simulink model "MOCS_AS_Gen"  (R2022b)
settings: Solver=FixedStepDiscrete  StartTime=0.0  StopTime=inf  FixedStep=0.1  RelTol=1e-3
undefined symbols (not defined in the file): CommonReservedCat2_typ, FODS_typ, FODSFeedback_typ, FODSFeedforward_typ, IF_PARA_CFlag, IF_PARA_CFODS, IF_PARA_CMain, IF_PARA_CReserved, IF_PARA_CSys, IF_PARA_No1FB, IF_PARA_No1FF, IF_PARA_No1Reserved, IF_PARA_No2FB, IF_PARA_No2FF, IF_PARA_No2Reserved, IF_PARA_No3FB, IF_PARA_No3FF, IF_PARA_No3Reserved, IF_PARA_No4FB, IF_PARA_No4FF, IF_PARA_No4Reserved, IF_PARA_No5FB, IF_PARA_No5FF, IF_PARA_No5Reserved, IF_PARA_No6FB, IF_PARA_No6FF, IF_PARA_No6Reserved, IF_PARA_No7FB, IF_PARA_No7FF, IF_PARA_No7Reserved, IF_PARA_No8FB, IF_PARA_No8FF, IF_PARA_No8Reserved, IndivReservedCat2_typ, Main_typ, StateFlag_typ, System_typ
libraries: bur_blks x39
settings Model: Creator=HHI  LastModifiedBy=HHI
settings DataIOCC: SaveFormat=Array  SaveOutput=off  SignalLogging=off  DSMLogging=off  SaveTime=off  ReturnWorkspaceOutputs=off
settings OptimizationCC: EnableMemcpy=off  ZeroExternalMemoryAtStartup=off  ZeroInternalMemoryAtStartup=off  InitFltsAndDblsToZero=on  LifeSpan=inf  OptimizeBlockOrder=speed  DifferentSizesBufferReuse=on  EfficientTunableParamExpr=on
settings DebuggingCC: UnderspecifiedInitializationDetection=Classic  MergeDetectMultiDrivingBlocksExec=none  SolverPrmCheckMsg=warning  InheritedTsInSrcMsg=none  FcnCallInpInsideContextMsg=warning  UnconnectedInputMsg=warning  UnconnectedOutputMsg=warning  UnconnectedLineMsg=warning  FrameProcessingCompatibilityMsg=none  ModelReferenceSymbolNameMessage=none  StateNameClashWarn=warning  SFUnexpectedBacktrackingDiag=warning  SFNoUnconditionalDefaultTransitionDiag=warning
settings HardwareCC: ProdBitPerPointer=32  ProdBitPerSizeT=32  ProdBitPerPtrDiffT=32  ProdLargestAtomicFloat=None  ProdWordSize=32  ProdHWDeviceType=Intel->x86/Pentium
settings ModelReferenceCC: UpdateModelReferenceTargets=IfOutOfDate  ModelReferencePassRootInputsByReference=off  PropagateSignalLabelsOutOfModel=off
settings SFSimCC: MATLABDynamicMemAlloc=off
settings RTWCC: Description=B&R Automation Studio Target (ERT based)  SystemTargetFile=bur_ert.tlc  GenCodeOnly=on  GenerateMakefile=off  TemplateMakefile=bur.tmf  RTWVerbose=off
settings CodeAppCC: IgnoreTestpoints=on  CustomSymbolStrType=$N$R$M  InternalIdentifier=Classic
settings STFCustomTargetCC: TargetLangStandard=C99 (ISO)  MultiwordLength=256  ParMdlRefBuildCompliant=on  ERTCustomFileBanners=on  SupportNonFinite=off  SupportNonInlinedSFcns=off  RemoveResetFunc=on  MATLABClassNameForMDSCustomization=Simulink.SoftwareTarget.ERTCustomization  SystemTargetFile=bur_ert.tlc
settings ERTTargetCC: TargetLangStandard=C99 (ISO)  CompOptLevelCompliant=off  ConcurrentExecutionCompliant=off  CombineOutputUpdateFcns=off  SupportNonFinite=off  SupportContinuousTime=on  ModelStepFunctionPrototypeControlCompliant=off  CPPClassGenCompliant=off  UseToolchainInfoCompliant=off  ExtModeMexArgs='127.0.0.1'  MultiInstanceErrorCode=Warning  RootIOFormat=Structure reference  ERTSrcFileBannerTemplate=bur_code_c_template.cgt  ERTHdrFileBannerTemplate=bur_code_h_template.cgt  ERTDataSrcFileTemplate=bur_data_c_template.cgt  ERTDataHdrFileTemplate=bur_data_h_template.cgt  ERTCustomFileTemplate=bur_file_process.tlc  ConvertIfToSwitch=off  SuppressUnreachableDefaultCases=off

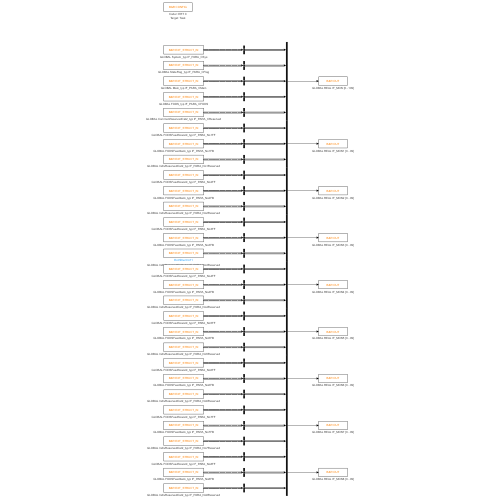
[thumbnail: Simulink's stored preview of the top-level diagram]
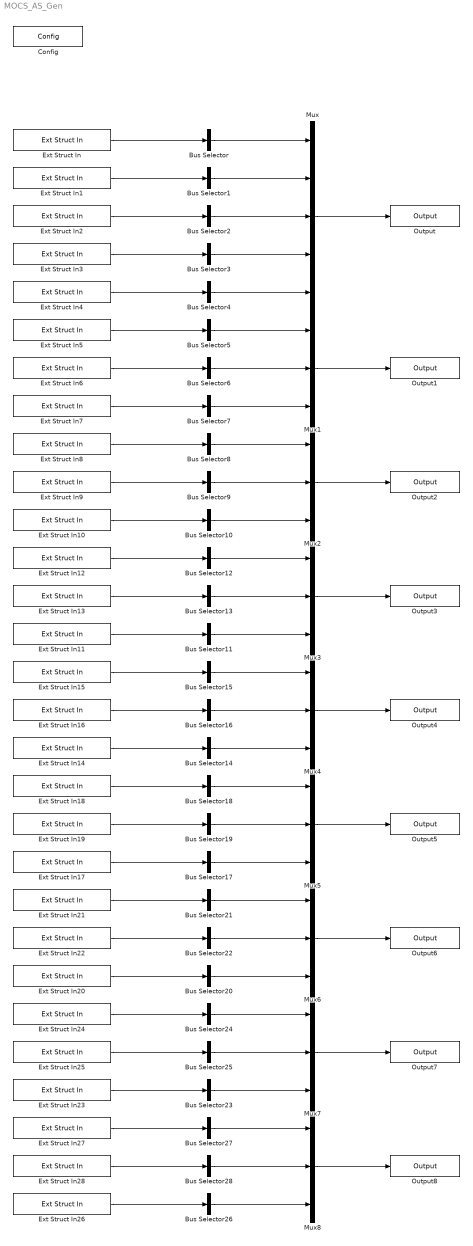
== system MOCS_AS_Gen ==
  Bus Selector : BusSelector  OutputSignals=SystemType.MOCSType,SystemType.NumofGE,SystemType.HeatingSystem,SystemType.FOSuppUnit,SystemReserved.SystemReserved4,SystemReserved.SystemReserved5,SystemReserved.SystemReserved6,SystemReserved.SystemReserved7,SystemReserved.SystemReserved8,SystemReserved.SystemReserved9,SystemReserved.SystemReserved10,SystemReserved.SystemReserved11,SystemReserved.SystemReserved12,SystemReserved.SystemReserved13,SystemReserved.SystemReserved14,SystemReserved.SystemReserved15,SystemReserved.SystemReserved16,SystemReserved.SystemReserved17,SystemReserved.SystemReserved18,SystemReserved.SystemReserved19,SystemReserved.SystemReserved20,SystemReserved.SystemReserved21,SystemReserved.SystemReserved22,SystemReserved.SystemReserved23,SystemReserved.SystemReserved24,SystemReserved.SystemReserved25,SystemReserved.SystemReserved26,SystemReserved.SystemReserved27,SystemReserved.SystemReserved28,SystemReserved.SystemReserved29,SystemReserved.SystemReserved30,SystemReserved.SystemReserved31,SystemReserved.SystemReserved32,SystemReserved.SystemReserved33,SystemReserved.SystemReserved34,SystemReserved.SystemReserved35,SystemReserved.SystemReserved36,SystemReserved.SystemReserved37,SystemReserved.SystemReserved38,SystemReserved.SystemReserved39,SystemReserved.SystemReserved40,SystemReserved.SystemReserved41,SystemReserved.SystemReserved42,SystemReserved.SystemReserved43,SystemReserved.SystemReserved44,SystemReserved.SystemReserved45,SystemReserved.SystemReserved46,SystemReserved.SystemReserved47,SystemReserved.SystemReserved48,SystemReserved.SystemReserved49  OutputAsBus=on
  Bus Selector1 : BusSelector  OutputSignals=MSSNormalFlag.MOCSMinEngineLoad,MSSNormalFlag.MOCSReadyEngineLoad,MSSNormalFlag.MSSNormalFallingHysteresis,MSSNormalFlag.MSSNormalFallingDelay,MSSNormalFlag.MSSFlagReserved4,LoadChangeFlag.MovAvgPeriod,LoadChangeFlag.ComparePoint,LoadChangeFlag.LoadChangeThreshold,LoadChangeFlag.TMBFlagFallingDelay,LoadChangeFlag.TMBFlagReserved4,SystemWarmedUpFlag.WarmUpDTemp,SystemWarmedUpFlag.WarmUpITemp,SystemWarmedUpFlag.WarmUpChITemp,SystemWarmedUpFlag.WarmUpChMTemp,SystemWarmedUpFlag.WarmUpChOTemp,FlagReserved.FlagReserved15,FlagReserved.FlagReserved16,FlagReserved.FlagReserved17,FlagReserved.FlagReserved18,FlagReserved.FlagReserved19,FlagReserved.FlagReserved20,FlagReserved.FlagReserved21,FlagReserved.FlagReserved22,FlagReserved.FlagReserved23,FlagReserved.FlagReserved24,FlagReserved.FlagReserved25,FlagReserved.FlagReserved26,FlagReserved.FlagReserved27,FlagReserved.FlagReserved28,FlagReserved.FlagReserved29,FlagReserved.FlagReserved30,FlagReserved.FlagReserved31,FlagReserved.FlagReserved32,FlagReserved.FlagReserved33,FlagReserved.FlagReserved34,FlagReserved.FlagReserved35,FlagReserved.FlagReserved36,FlagReserved.FlagReserved37,FlagReserved.FlagReserved38,FlagReserved.FlagReserved39,FlagReserved.FlagReserved40,FlagReserved.FlagReserved41,FlagReserved.FlagReserved42,FlagReserved.FlagReserved43,FlagReserved.FlagReserved44,FlagReserved.FlagReserved45,FlagReserved.FlagReserved46,FlagReserved.FlagReserved47,FlagReserved.FlagReserved48,FlagReserved.FlagReserved49  OutputAsBus=on
  Bus Selector{7,10..11,14,17,20,23,26} (8 alike) : BusSelector  OutputSignals=IndivReservedCat3.IndivReserved75,IndivReservedCat3.IndivReserved76,IndivReservedCat3.IndivReserved77,IndivReservedCat3.IndivReserved78,IndivReservedCat3.IndivReserved79,IndivReservedCat3.IndivReserved80,IndivReservedCat3.IndivReserved81,IndivReservedCat3.IndivReserved82,IndivReservedCat3.IndivReserved83,IndivReservedCat3.IndivReserved84,IndivReservedCat3.IndivReserved85,IndivReservedCat3.IndivReserved86,IndivReservedCat3.IndivReserved87,IndivReservedCat3.IndivReserved88,IndivReservedCat3.IndivReserved89,IndivReservedCat3.IndivReserved90,IndivReservedCat3.IndivReserved91,IndivReservedCat3.IndivReserved92,IndivReservedCat3.IndivReserved93,IndivReservedCat3.IndivReserved94,IndivReservedCat3.IndivReserved95,IndivReservedCat3.IndivReserved96,IndivReservedCat3.IndivReserved97,IndivReservedCat3.IndivReserved98,IndivReservedCat3.IndivReserved99  OutputAsBus=on
  Bus Selector{5,8,12,15,18,21,24,27} (8 alike) : BusSelector  OutputSignals=FFpara.NumTableRow,FFpara.HeatLossTemp,EngineLoad.EngineLoad0,EngineLoad.EngineLoad1,EngineLoad.EngineLoad2,EngineLoad.EngineLoad3,EngineLoad.EngineLoad4,EngineLoad.EngineLoad5,EngineLoad.EngineLoad6,EngineLoad.EngineLoad7,EngineLoad.EngineLoad8,EngineLoad.EngineLoad9,EngineLoad.EngineLoad10,EngineLoad.EngineLoad11,ExhFlowrate.ExhFlowrate0,ExhFlowrate.ExhFlowrate1,ExhFlowrate.ExhFlowrate2,ExhFlowrate.ExhFlowrate3,ExhFlowrate.ExhFlowrate4,ExhFlowrate.ExhFlowrate5,ExhFlowrate.ExhFlowrate6,ExhFlowrate.ExhFlowrate7,ExhFlowrate.ExhFlowrate8,ExhFlowrate.ExhFlowrate9,ExhFlowrate.ExhFlowrate10,ExhFlowrate.ExhFlowrate11,HUInletRefTemp.HUInletRefTemp0,HUInletRefTemp.HUInletRefTemp1,HUInletRefTemp.HUInletRefTemp2,HUInletRefTemp.HUInletRefTemp3,HUInletRefTemp.HUInletRefTemp4,HUInletRefTemp.HUInletRefTemp5,HUInletRefTemp.HUInletRefTemp6,HUInletRefTemp.HUInletRefTemp7,HUInletRefTemp.HUInletRefTemp8,HUInletRefTemp.HUInletRefTemp9,HUInletRefTemp.HUInletRefTemp10,HUInletRefTemp.HUInletRefTemp11,CorrectionFactor.CorrectionFactor0,CorrectionFactor.CorrectionFactor1,CorrectionFactor.CorrectionFactor2,CorrectionFactor.CorrectionFactor3,CorrectionFactor.CorrectionFactor4,CorrectionFactor.CorrectionFactor5,CorrectionFactor.CorrectionFactor6,CorrectionFactor.CorrectionFactor7,CorrectionFactor.CorrectionFactor8,CorrectionFactor.CorrectionFactor9,CorrectionFactor.CorrectionFactor10,CorrectionFactor.CorrectionFactor11  OutputAsBus=on
  Bus Selector{6,9,13,16,19,22,25,28} (8 alike) : BusSelector  OutputSignals=MOCSTempPgain.MOCSTempPgain0,MOCSTempPgain.MOCSTempPgain1,MOCSTempPgain.MOCSTempPgain2,MOCSTempPgain.MOCSTempPgain3,MOCSTempPgain.MOCSTempPgain4,MOCSTempPgain.MOCSTempPgain5,MOCSTempPgain.MOCSTempPgain6,MOCSTempPgain.MOCSTempPgain7,MOCSTempPgain.MOCSTempPgain8,MOCSTempPgain.MOCSTempPgain9,MOCSTempPgain.MOCSTempPgain10,MOCSTempPgain.MOCSTempPgain11,APIDgain.MOCSTempIgain,APIDgain.MOCSTempDgain,APIDgain.MOCSTempNoiseSup,APIDgain.QFOPgain,APIDgain.QFOIgain,APIDgain.QFODgain,APIDgain.QFONoiseSup,APIDgain.FODSFeedbackReserved19,APIDgain.FODSFeedbackReserved20,APIDgain.FODSFeedbackReserved21,APIDgain.FODSFeedbackReserved22,APIDgain.FODSFeedbackReserved23,APIDgain.FODSFeedbackReserved24  OutputAsBus=on
  Bus Selector2 : BusSelector  OutputSignals=Init.InitReserved0,Init.InitReserved1,Init.InitReserved2,Init.InitReserved3,Init.InitReserved4,Sealing.VSSolValveOpenDP,Sealing.VSSolValveCloseDP,Sealing.RTVOpenDP,Sealing.RTVCloseDP,Sealing.SealRTVSetpoint,Sealing.VSSolValveOpenDuration,Sealing.VSSolValveCloseDuration,Sealing.SealingReserved7,Sealing.SealingReserved8,Sealing.SealingReserved9,Engage.EnRTVSlope,Engage.EngageReserved1,Engage.EngageReserved2,Engage.EngageReserved3,Engage.EngageReserved4,Active.HUTargetTemp,Active.HUActiveTemp,Active.HUInactiveOffsetTemp,Active.ActiveReserved3,Active.ActiveReserved4,TMB.TMBBypassMinDuration,TMB.TMBTimeoutThreshold,TMB.TMBReserved2,TMB.TMBReserved3,TMB.TMBReserved4,Disengage.DisenRTVSlope,Disengage.DisengageReserved1,Disengage.DisengageReserved2,Disengage.DisengageReserved3,Disengage.DisengageReserved4,Airventing.VentRTVSetpoint,Airventing.VentDuration,Airventing.AirVentingReserved2,Airventing.AirVentingReserved3,Airventing.AirVentingReserved4,MOCSshutdown.MOCSShutdownReserved0,MOCSshutdown.MOCSShutdownReserved1,MOCSshutdown.MOCSShutdownReserved2,MOCSshutdown.MOCSShutdownReserved3,MOCSshutdown.MOCSShutdownReserved4,Valveshutdown.ValveShutdownReserved0,Valveshutdown.ValveShutdownReserved1,Valveshutdown.ValveShutdownReserved2,Valveshutdown.ValveShutdownReserved3,Valveshutdown.ValveShutdownReserved4  OutputAsBus=on
  Bus Selector3 : BusSelector  OutputSignals=FODSInitReady.FODSInitReserved0,FODSInitReady.FODSInitReserved1,FODSInitReady.FODSInitReserved2,FODSInitReady.FODSInitReserved3,FODSInitReady.FODSInitReserved4,FODSCooling.FOCoolDuration,FODSCooling.FODSCoolingReserved1,FODSCooling.FODSCoolingReserved2,FODSCooling.FODSCoolingReserved3,FODSCooling.FODSCoolingReserved4,FODSDosing.PumpChangeOverTime,FODSDosing.SolVVDelay,FODSDosing.LowRefQFOTimeout,FODSDosing.QFOLowLimitTimeout,FODSDosing.SFFlowrateThHigh,FODSDosing.SFFlowrateThLow,FODSDosing.QFOHighLimitGain,FODSDosing.QFOHighLimitMin,FODSDosing.QFOLowLimitValue,FODSDosing.FOCValHighLimitValue,FODSDosing.FOCValLowLimitValue,FODSDosing.FODSDosingReserved11,FODSDosing.FODSDosingReserved12,FODSDosing.FODSDosingReserved13,FODSDosing.FODSDosingReserved14,FODSFlushing.FOReturnDelay,FODSFlushing.FOPurgingDuration,FODSFlushing.FODSFlushingReserved2,FODSFlushing.FODSFlushingReserved3,FODSFlushing.FODSFlushingReserved4  OutputAsBus=on
  Bus Selector4 : BusSelector  OutputSignals=CommonReservedCat3.CommReserved180,CommonReservedCat3.CommReserved181,CommonReservedCat3.CommReserved182,CommonReservedCat3.CommReserved183,CommonReservedCat3.CommReserved184,CommonReservedCat3.CommReserved185,CommonReservedCat3.CommReserved186,CommonReservedCat3.CommReserved187,CommonReservedCat3.CommReserved188,CommonReservedCat3.CommReserved189,CommonReservedCat3.CommReserved190,CommonReservedCat3.CommReserved191,CommonReservedCat3.CommReserved192,CommonReservedCat3.CommReserved193,CommonReservedCat3.CommReserved194,CommonReservedCat3.CommReserved195,CommonReservedCat3.CommReserved196,CommonReservedCat3.CommReserved197,CommonReservedCat3.CommReserved198,CommonReservedCat3.CommReserved199  OutputAsBus=on
  Config : bur_blks/Config  Tag=Coder: ERT C Target: Task  bur_configset_ert=C - Code Generation (Embedded Real Time Target based)  bur_configset_grt=C - Code Generation (Generic Real Time Target based)  bur_maskHandle=-1
      settings: AttributesFormatString=%<Tag>  SourceProductName=B&R Automation Studio Toolbox
  Ext Struct In : bur_blks/Ext Struct In  Tag=GLOBAL System_typ IF_PARA_CSys  bur_var_name=IF_PARA_CSys  bur_scope=GLOBAL  bur_var_memory=standard  bur_struct_name=System_typ  bur_AS_string=IF_PARA_CSys : System_typ; (**)  bur_AS_typ_list_string=|
      | System_typ
      | Bus: SystemType_typ
      | Bus: SystemReserved_typ
      settings: AttributesFormatString=%<Tag>  SourceProductName=B&R Automation Studio Toolbox
  Ext Struct In1 : bur_blks/Ext Struct In  Tag=GLOBAL StateFlag_typ IF_PARA_CFlag  bur_var_name=IF_PARA_CFlag  bur_scope=GLOBAL  bur_var_memory=standard  bur_struct_name=StateFlag_typ  bur_AS_string=IF_PARA_CFlag : StateFlag_typ; (**)  bur_AS_typ_list_string=|
      | StateFlag_typ
      | Bus: MSSNormalFlag_typ
      | Bus: LoadChangeFlag_typ
      | Bus: SystemWarmedUpFlag_typ
      | Bus: FlagReserved_typ
      settings: AttributesFormatString=%<Tag>  SourceProductName=B&R Automation Studio Toolbox
  Ext Struct In10 : bur_blks/Ext Struct In  Tag=GLOBAL IndivReservedCat2_typ IF_PARA_No2Reserved  bur_var_name=IF_PARA_No2Reserved  bur_scope=GLOBAL  bur_var_memory=standard  bur_struct_name=IndivReservedCat2_typ  bur_AS_string=IF_PARA_No2Reserved : IndivReservedCat2_typ; (**)  bur_AS_typ_list_string=IndivReservedCat2_typ Bus: IndivReservedCat3_typ
      settings: AttributesFormatString=%<Tag>  SourceProductName=B&R Automation Studio Toolbox
  Ext Struct In11 : bur_blks/Ext Struct In  Tag=GLOBAL IndivReservedCat2_typ IF_PARA_No3Reserved  bur_var_name=IF_PARA_No3Reserved  bur_scope=GLOBAL  bur_var_memory=standard  bur_struct_name=IndivReservedCat2_typ  bur_AS_string=IF_PARA_No3Reserved : IndivReservedCat2_typ; (**)  bur_AS_typ_list_string=IndivReservedCat2_typ Bus: IndivReservedCat3_typ
      settings: AttributesFormatString=%<Tag>  SourceProductName=B&R Automation Studio Toolbox
  Ext Struct In12 : bur_blks/Ext Struct In  Tag=GLOBAL FODSFeedforward_typ IF_PARA_No3FF  bur_var_name=IF_PARA_No3FF  bur_scope=GLOBAL  bur_var_memory=standard  bur_struct_name=FODSFeedforward_typ  bur_AS_string=IF_PARA_No3FF : FODSFeedforward_typ; (**)  bur_AS_typ_list_string=|
      | FODSFeedforward_typ
      | Bus: FFpara_typ
      | Bus: EngineLoad_typ
      | Bus: ExhFlowrate_typ
      | Bus: HUInletRefTemp_typ
      | Bus: CorrectionFactor_typ
      settings: AttributesFormatString=%<Tag>  SourceProductName=B&R Automation Studio Toolbox
  Ext Struct In13 : bur_blks/Ext Struct In  Tag=GLOBAL FODSFeedback_typ IF_PARA_No3FB  bur_var_name=IF_PARA_No3FB  bur_scope=GLOBAL  bur_var_memory=standard  bur_struct_name=FODSFeedback_typ  bur_AS_string=IF_PARA_No3FB : FODSFeedback_typ; (**)  bur_AS_typ_list_string=|
      | FODSFeedback_typ
      | Bus: MOCSTempPgain_typ
      | Bus: APIDgain_typ
      settings: AttributesFormatString=%<Tag>  SourceProductName=B&R Automation Studio Toolbox
  Ext Struct In14 : bur_blks/Ext Struct In  Tag=GLOBAL IndivReservedCat2_typ IF_PARA_No4Reserved  bur_var_name=IF_PARA_No4Reserved  bur_scope=GLOBAL  bur_var_memory=standard  bur_struct_name=IndivReservedCat2_typ  bur_AS_string=IF_PARA_No4Reserved : IndivReservedCat2_typ; (**)  bur_AS_typ_list_string=IndivReservedCat2_typ Bus: IndivReservedCat3_typ
      settings: AttributesFormatString=%<Tag>  SourceProductName=B&R Automation Studio Toolbox
  Ext Struct In15 : bur_blks/Ext Struct In  Tag=GLOBAL FODSFeedforward_typ IF_PARA_No4FF  bur_var_name=IF_PARA_No4FF  bur_scope=GLOBAL  bur_var_memory=standard  bur_struct_name=FODSFeedforward_typ  bur_AS_string=IF_PARA_No4FF : FODSFeedforward_typ; (**)  bur_AS_typ_list_string=|
      | FODSFeedforward_typ
      | Bus: FFpara_typ
      | Bus: EngineLoad_typ
      | Bus: ExhFlowrate_typ
      | Bus: HUInletRefTemp_typ
      | Bus: CorrectionFactor_typ
      settings: AttributesFormatString=%<Tag>  SourceProductName=B&R Automation Studio Toolbox
  Ext Struct In16 : bur_blks/Ext Struct In  Tag=GLOBAL FODSFeedback_typ IF_PARA_No4FB  bur_var_name=IF_PARA_No4FB  bur_scope=GLOBAL  bur_var_memory=standard  bur_struct_name=FODSFeedback_typ  bur_AS_string=IF_PARA_No4FB : FODSFeedback_typ; (**)  bur_AS_typ_list_string=|
      | FODSFeedback_typ
      | Bus: MOCSTempPgain_typ
      | Bus: APIDgain_typ
      settings: AttributesFormatString=%<Tag>  SourceProductName=B&R Automation Studio Toolbox
  Ext Struct In17 : bur_blks/Ext Struct In  Tag=GLOBAL IndivReservedCat2_typ IF_PARA_No5Reserved  bur_var_name=IF_PARA_No5Reserved  bur_scope=GLOBAL  bur_var_memory=standard  bur_struct_name=IndivReservedCat2_typ  bur_AS_string=IF_PARA_No5Reserved : IndivReservedCat2_typ; (**)  bur_AS_typ_list_string=IndivReservedCat2_typ Bus: IndivReservedCat3_typ
      settings: AttributesFormatString=%<Tag>  SourceProductName=B&R Automation Studio Toolbox
  Ext Struct In18 : bur_blks/Ext Struct In  Tag=GLOBAL FODSFeedforward_typ IF_PARA_No5FF  bur_var_name=IF_PARA_No5FF  bur_scope=GLOBAL  bur_var_memory=standard  bur_struct_name=FODSFeedforward_typ  bur_AS_string=IF_PARA_No5FF : FODSFeedforward_typ; (**)  bur_AS_typ_list_string=|
      | FODSFeedforward_typ
      | Bus: FFpara_typ
      | Bus: EngineLoad_typ
      | Bus: ExhFlowrate_typ
      | Bus: HUInletRefTemp_typ
      | Bus: CorrectionFactor_typ
      settings: AttributesFormatString=%<Tag>  SourceProductName=B&R Automation Studio Toolbox
  Ext Struct In19 : bur_blks/Ext Struct In  Tag=GLOBAL FODSFeedback_typ IF_PARA_No5FB  bur_var_name=IF_PARA_No5FB  bur_scope=GLOBAL  bur_var_memory=standard  bur_struct_name=FODSFeedback_typ  bur_AS_string=IF_PARA_No5FB : FODSFeedback_typ; (**)  bur_AS_typ_list_string=|
      | FODSFeedback_typ
      | Bus: MOCSTempPgain_typ
      | Bus: APIDgain_typ
      settings: AttributesFormatString=%<Tag>  SourceProductName=B&R Automation Studio Toolbox
  Ext Struct In2 : bur_blks/Ext Struct In  Tag=GLOBAL Main_typ IF_PARA_CMain  bur_var_name=IF_PARA_CMain  bur_scope=GLOBAL  bur_var_memory=standard  bur_struct_name=Main_typ  bur_AS_string=IF_PARA_CMain : Main_typ; (**)  bur_AS_typ_list_string=|
      | Main_typ
      | Bus: Init_typ
      | Bus: Sealing_typ
      | Bus: Engage_typ
      | Bus: Active_typ
      | Bus: TMB_typ
      | Bus: Disengage_typ
      | Bus: Airventing_typ
      | Bus: MOCSshutdown_typ
      | Bus: Valveshutdown_typ
      settings: AttributesFormatString=%<Tag>  SourceProductName=B&R Automation Studio Toolbox
  Ext Struct In20 : bur_blks/Ext Struct In  Tag=GLOBAL IndivReservedCat2_typ IF_PARA_No6Reserved  bur_var_name=IF_PARA_No6Reserved  bur_scope=GLOBAL  bur_var_memory=standard  bur_struct_name=IndivReservedCat2_typ  bur_AS_string=IF_PARA_No6Reserved : IndivReservedCat2_typ; (**)  bur_AS_typ_list_string=IndivReservedCat2_typ Bus: IndivReservedCat3_typ
      settings: AttributesFormatString=%<Tag>  SourceProductName=B&R Automation Studio Toolbox
  Ext Struct In21 : bur_blks/Ext Struct In  Tag=GLOBAL FODSFeedforward_typ IF_PARA_No6FF  bur_var_name=IF_PARA_No6FF  bur_scope=GLOBAL  bur_var_memory=standard  bur_struct_name=FODSFeedforward_typ  bur_AS_string=IF_PARA_No6FF : FODSFeedforward_typ; (**)  bur_AS_typ_list_string=|
      | FODSFeedforward_typ
      | Bus: FFpara_typ
      | Bus: EngineLoad_typ
      | Bus: ExhFlowrate_typ
      | Bus: HUInletRefTemp_typ
      | Bus: CorrectionFactor_typ
      settings: AttributesFormatString=%<Tag>  SourceProductName=B&R Automation Studio Toolbox
  Ext Struct In22 : bur_blks/Ext Struct In  Tag=GLOBAL FODSFeedback_typ IF_PARA_No6FB  bur_var_name=IF_PARA_No6FB  bur_scope=GLOBAL  bur_var_memory=standard  bur_struct_name=FODSFeedback_typ  bur_AS_string=IF_PARA_No6FB : FODSFeedback_typ; (**)  bur_AS_typ_list_string=|
      | FODSFeedback_typ
      | Bus: MOCSTempPgain_typ
      | Bus: APIDgain_typ
      settings: AttributesFormatString=%<Tag>  SourceProductName=B&R Automation Studio Toolbox
  Ext Struct In23 : bur_blks/Ext Struct In  Tag=GLOBAL IndivReservedCat2_typ IF_PARA_No7Reserved  bur_var_name=IF_PARA_No7Reserved  bur_scope=GLOBAL  bur_var_memory=standard  bur_struct_name=IndivReservedCat2_typ  bur_AS_string=IF_PARA_No7Reserved : IndivReservedCat2_typ; (**)  bur_AS_typ_list_string=IndivReservedCat2_typ Bus: IndivReservedCat3_typ
      settings: AttributesFormatString=%<Tag>  SourceProductName=B&R Automation Studio Toolbox
  Ext Struct In24 : bur_blks/Ext Struct In  Tag=GLOBAL FODSFeedforward_typ IF_PARA_No7FF  bur_var_name=IF_PARA_No7FF  bur_scope=GLOBAL  bur_var_memory=standard  bur_struct_name=FODSFeedforward_typ  bur_AS_string=IF_PARA_No7FF : FODSFeedforward_typ; (**)  bur_AS_typ_list_string=|
      | FODSFeedforward_typ
      | Bus: FFpara_typ
      | Bus: EngineLoad_typ
      | Bus: ExhFlowrate_typ
      | Bus: HUInletRefTemp_typ
      | Bus: CorrectionFactor_typ
      settings: AttributesFormatString=%<Tag>  SourceProductName=B&R Automation Studio Toolbox
  Ext Struct In25 : bur_blks/Ext Struct In  Tag=GLOBAL FODSFeedback_typ IF_PARA_No7FB  bur_var_name=IF_PARA_No7FB  bur_scope=GLOBAL  bur_var_memory=standard  bur_struct_name=FODSFeedback_typ  bur_AS_string=IF_PARA_No7FB : FODSFeedback_typ; (**)  bur_AS_typ_list_string=|
      | FODSFeedback_typ
      | Bus: MOCSTempPgain_typ
      | Bus: APIDgain_typ
      settings: AttributesFormatString=%<Tag>  SourceProductName=B&R Automation Studio Toolbox
  Ext Struct In26 : bur_blks/Ext Struct In  Tag=GLOBAL IndivReservedCat2_typ IF_PARA_No8Reserved  bur_var_name=IF_PARA_No8Reserved  bur_scope=GLOBAL  bur_var_memory=standard  bur_struct_name=IndivReservedCat2_typ  bur_AS_string=IF_PARA_No8Reserved : IndivReservedCat2_typ; (**)  bur_AS_typ_list_string=IndivReservedCat2_typ Bus: IndivReservedCat3_typ
      settings: AttributesFormatString=%<Tag>  SourceProductName=B&R Automation Studio Toolbox
  Ext Struct In27 : bur_blks/Ext Struct In  Tag=GLOBAL FODSFeedforward_typ IF_PARA_No8FF  bur_var_name=IF_PARA_No8FF  bur_scope=GLOBAL  bur_var_memory=standard  bur_struct_name=FODSFeedforward_typ  bur_AS_string=IF_PARA_No8FF : FODSFeedforward_typ; (**)  bur_AS_typ_list_string=|
      | FODSFeedforward_typ
      | Bus: FFpara_typ
      | Bus: EngineLoad_typ
      | Bus: ExhFlowrate_typ
      | Bus: HUInletRefTemp_typ
      | Bus: CorrectionFactor_typ
      settings: AttributesFormatString=%<Tag>  SourceProductName=B&R Automation Studio Toolbox
  Ext Struct In28 : bur_blks/Ext Struct In  Tag=GLOBAL FODSFeedback_typ IF_PARA_No8FB  bur_var_name=IF_PARA_No8FB  bur_scope=GLOBAL  bur_var_memory=standard  bur_struct_name=FODSFeedback_typ  bur_AS_string=IF_PARA_No8FB : FODSFeedback_typ; (**)  bur_AS_typ_list_string=|
      | FODSFeedback_typ
      | Bus: MOCSTempPgain_typ
      | Bus: APIDgain_typ
      settings: AttributesFormatString=%<Tag>  SourceProductName=B&R Automation Studio Toolbox
  Ext Struct In3 : bur_blks/Ext Struct In  Tag=GLOBAL FODS_typ IF_PARA_CFODS  bur_var_name=IF_PARA_CFODS  bur_scope=GLOBAL  bur_var_memory=standard  bur_struct_name=FODS_typ  bur_AS_string=IF_PARA_CFODS : FODS_typ; (**)  bur_AS_typ_list_string=|
      | FODS_typ
      | Bus: FODSInitReady_typ
      | Bus: FODSCooling_typ
      | Bus: FODSDosing_typ
      | Bus: FODSFlushing_typ
      settings: AttributesFormatString=%<Tag>  SourceProductName=B&R Automation Studio Toolbox
  Ext Struct In4 : bur_blks/Ext Struct In  Tag=GLOBAL CommonReservedCat2_typ IF_PARA_CReserved  bur_var_name=IF_PARA_CReserved  bur_scope=GLOBAL  bur_var_memory=standard  bur_struct_name=CommonReservedCat2_typ  bur_AS_string=IF_PARA_CReserved : CommonReservedCat2_typ; (**)  bur_AS_typ_list_string=CommonReservedCat2_typ Bus: CommonReservedCat3_typ
      settings: AttributesFormatString=%<Tag>  SourceProductName=B&R Automation Studio Toolbox
  Ext Struct In5 : bur_blks/Ext Struct In  Tag=GLOBAL FODSFeedforward_typ IF_PARA_No1FF  bur_var_name=IF_PARA_No1FF  bur_scope=GLOBAL  bur_var_memory=standard  bur_struct_name=FODSFeedforward_typ  bur_AS_string=IF_PARA_No1FF : FODSFeedforward_typ; (**)  bur_AS_typ_list_string=|
      | FODSFeedforward_typ
      | Bus: FFpara_typ
      | Bus: EngineLoad_typ
      | Bus: ExhFlowrate_typ
      | Bus: HUInletRefTemp_typ
      | Bus: CorrectionFactor_typ
      settings: AttributesFormatString=%<Tag>  SourceProductName=B&R Automation Studio Toolbox
  Ext Struct In6 : bur_blks/Ext Struct In  Tag=GLOBAL FODSFeedback_typ IF_PARA_No1FB  bur_var_name=IF_PARA_No1FB  bur_scope=GLOBAL  bur_var_memory=standard  bur_struct_name=FODSFeedback_typ  bur_AS_string=IF_PARA_No1FB : FODSFeedback_typ; (**)  bur_AS_typ_list_string=|
      | FODSFeedback_typ
      | Bus: MOCSTempPgain_typ
      | Bus: APIDgain_typ
      settings: AttributesFormatString=%<Tag>  SourceProductName=B&R Automation Studio Toolbox
  Ext Struct In7 : bur_blks/Ext Struct In  Tag=GLOBAL IndivReservedCat2_typ IF_PARA_No1Reserved  bur_var_name=IF_PARA_No1Reserved  bur_scope=GLOBAL  bur_var_memory=standard  bur_struct_name=IndivReservedCat2_typ  bur_AS_string=IF_PARA_No1Reserved : IndivReservedCat2_typ; (**)  bur_AS_typ_list_string=IndivReservedCat2_typ Bus: IndivReservedCat3_typ
      settings: AttributesFormatString=%<Tag>  SourceProductName=B&R Automation Studio Toolbox
  Ext Struct In8 : bur_blks/Ext Struct In  Tag=GLOBAL FODSFeedforward_typ IF_PARA_No2FF  bur_var_name=IF_PARA_No2FF  bur_scope=GLOBAL  bur_var_memory=standard  bur_struct_name=FODSFeedforward_typ  bur_AS_string=IF_PARA_No2FF : FODSFeedforward_typ; (**)  bur_AS_typ_list_string=|
      | FODSFeedforward_typ
      | Bus: FFpara_typ
      | Bus: EngineLoad_typ
      | Bus: ExhFlowrate_typ
      | Bus: HUInletRefTemp_typ
      | Bus: CorrectionFactor_typ
      settings: AttributesFormatString=%<Tag>  SourceProductName=B&R Automation Studio Toolbox
  Ext Struct In9 : bur_blks/Ext Struct In  Tag=GLOBAL FODSFeedback_typ IF_PARA_No2FB  bur_var_name=IF_PARA_No2FB  bur_scope=GLOBAL  bur_var_memory=standard  bur_struct_name=FODSFeedback_typ  bur_AS_string=IF_PARA_No2FB : FODSFeedback_typ; (**)  bur_AS_typ_list_string=|
      | FODSFeedback_typ
      | Bus: MOCSTempPgain_typ
      | Bus: APIDgain_typ
      settings: AttributesFormatString=%<Tag>  SourceProductName=B&R Automation Studio Toolbox
  Mux : Mux  Inputs=5
  Mux{1..8} (8 alike) : Mux  Inputs=3
  Output : bur_blks/Output  Tag=GLOBAL REAL IF_MON [0...199]  bur_var_name=IF_MON  bur_scope=GLOBAL  bur_data_type=REAL  bur_init_value=0  bur_init_value_bool=FALSE  bur_array_index=199  bur_var_memory=standard  bur_AS_string=IF_MON : ARRAY[0..199] OF REAL:= [200(0)]; (**)  bur_array_index_string=199
      settings: AttributesFormatString=%<Tag>  SourceProductName=B&R Automation Studio Toolbox
  Output1 : bur_blks/Output  Tag=GLOBAL REAL IF_MON1 [0...99]  bur_var_name=IF_MON1  bur_scope=GLOBAL  bur_data_type=REAL  bur_init_value=0  bur_init_value_bool=FALSE  bur_array_index=99  bur_var_memory=standard  bur_AS_string=IF_MON1 : ARRAY[0..99] OF REAL:= [100(0)]; (**)  bur_array_index_string=99
      settings: AttributesFormatString=%<Tag>  SourceProductName=B&R Automation Studio Toolbox
  Output2 : bur_blks/Output  Tag=GLOBAL REAL IF_MON2 [0...99]  bur_var_name=IF_MON2  bur_scope=GLOBAL  bur_data_type=REAL  bur_init_value=0  bur_init_value_bool=FALSE  bur_array_index=99  bur_var_memory=standard  bur_AS_string=IF_MON2 : ARRAY[0..99] OF REAL:= [100(0)]; (**)  bur_array_index_string=99
      settings: AttributesFormatString=%<Tag>  SourceProductName=B&R Automation Studio Toolbox
  Output3 : bur_blks/Output  Tag=GLOBAL REAL IF_MON3 [0...99]  bur_var_name=IF_MON3  bur_scope=GLOBAL  bur_data_type=REAL  bur_init_value=0  bur_init_value_bool=FALSE  bur_array_index=99  bur_var_memory=standard  bur_AS_string=IF_MON3 : ARRAY[0..99] OF REAL:= [100(0)]; (**)  bur_array_index_string=99
      settings: AttributesFormatString=%<Tag>  SourceProductName=B&R Automation Studio Toolbox
  Output4 : bur_blks/Output  Tag=GLOBAL REAL IF_MON4 [0...99]  bur_var_name=IF_MON4  bur_scope=GLOBAL  bur_data_type=REAL  bur_init_value=0  bur_init_value_bool=FALSE  bur_array_index=99  bur_var_memory=standard  bur_AS_string=IF_MON4 : ARRAY[0..99] OF REAL:= [100(0)]; (**)  bur_array_index_string=99
      settings: AttributesFormatString=%<Tag>  SourceProductName=B&R Automation Studio Toolbox
  Output5 : bur_blks/Output  Tag=GLOBAL REAL IF_MON5 [0...99]  bur_var_name=IF_MON5  bur_scope=GLOBAL  bur_data_type=REAL  bur_init_value=0  bur_init_value_bool=FALSE  bur_array_index=99  bur_var_memory=standard  bur_AS_string=IF_MON5 : ARRAY[0..99] OF REAL:= [100(0)]; (**)  bur_array_index_string=99
      settings: AttributesFormatString=%<Tag>  SourceProductName=B&R Automation Studio Toolbox
  Output6 : bur_blks/Output  Tag=GLOBAL REAL IF_MON6 [0...99]  bur_var_name=IF_MON6  bur_scope=GLOBAL  bur_data_type=REAL  bur_init_value=0  bur_init_value_bool=FALSE  bur_array_index=99  bur_var_memory=standard  bur_AS_string=IF_MON6 : ARRAY[0..99] OF REAL:= [100(0)]; (**)  bur_array_index_string=99
      settings: AttributesFormatString=%<Tag>  SourceProductName=B&R Automation Studio Toolbox
  Output7 : bur_blks/Output  Tag=GLOBAL REAL IF_MON7 [0...99]  bur_var_name=IF_MON7  bur_scope=GLOBAL  bur_data_type=REAL  bur_init_value=0  bur_init_value_bool=FALSE  bur_array_index=99  bur_var_memory=standard  bur_AS_string=IF_MON7 : ARRAY[0..99] OF REAL:= [100(0)]; (**)  bur_array_index_string=99
      settings: AttributesFormatString=%<Tag>  SourceProductName=B&R Automation Studio Toolbox
  Output8 : bur_blks/Output  Tag=GLOBAL REAL IF_MON8 [0...99]  bur_var_name=IF_MON8  bur_scope=GLOBAL  bur_data_type=REAL  bur_init_value=0  bur_init_value_bool=FALSE  bur_array_index=99  bur_var_memory=standard  bur_AS_string=IF_MON8 : ARRAY[0..99] OF REAL:= [100(0)]; (**)  bur_array_index_string=99
      settings: AttributesFormatString=%<Tag>  SourceProductName=B&R Automation Studio Toolbox
  wires:
  Ext Struct In/1 -> Bus Selector/1
  Bus Selector/1 -> Mux/1
  Bus Selector1/1 -> Mux/2
  Ext Struct In1/1 -> Bus Selector1/1
  Mux/1 -> Output/1
  Ext Struct In2/1 -> Bus Selector2/1
  Bus Selector2/1 -> Mux/3
  Ext Struct In3/1 -> Bus Selector3/1
  Bus Selector3/1 -> Mux/4
  Bus Selector4/1 -> Mux/5
  Ext Struct In4/1 -> Bus Selector4/1
  Bus Selector7/1 -> Mux1/3
  Ext Struct In7/1 -> Bus Selector7/1
  Mux1/1 -> Output1/1
  Ext Struct In6/1 -> Bus Selector6/1
  Bus Selector6/1 -> Mux1/2
  Bus Selector5/1 -> Mux1/1
  Ext Struct In5/1 -> Bus Selector5/1
  Ext Struct In8/1 -> Bus Selector8/1
  Bus Selector8/1 -> Mux2/1
  Bus Selector9/1 -> Mux2/2
  Ext Struct In9/1 -> Bus Selector9/1
  Mux2/1 -> Output2/1
  Ext Struct In10/1 -> Bus Selector10/1
  Bus Selector10/1 -> Mux2/3
  Bus Selector11/1 -> Mux3/3
  Ext Struct In11/1 -> Bus Selector11/1
  Mux3/1 -> Output3/1
  Ext Struct In13/1 -> Bus Selector13/1
  Bus Selector13/1 -> Mux3/2
  Bus Selector12/1 -> Mux3/1
  Ext Struct In12/1 -> Bus Selector12/1
  Ext Struct In15/1 -> Bus Selector15/1
  Bus Selector15/1 -> Mux4/1
  Bus Selector16/1 -> Mux4/2
  Ext Struct In16/1 -> Bus Selector16/1
  Mux4/1 -> Output4/1
  Ext Struct In14/1 -> Bus Selector14/1
  Bus Selector14/1 -> Mux4/3
  Bus Selector17/1 -> Mux5/3
  Ext Struct In17/1 -> Bus Selector17/1
  Mux5/1 -> Output5/1
  Ext Struct In19/1 -> Bus Selector19/1
  Bus Selector19/1 -> Mux5/2
  Bus Selector18/1 -> Mux5/1
  Ext Struct In18/1 -> Bus Selector18/1
  Ext Struct In21/1 -> Bus Selector21/1
  Bus Selector21/1 -> Mux6/1
  Bus Selector22/1 -> Mux6/2
  Ext Struct In22/1 -> Bus Selector22/1
  Mux6/1 -> Output6/1
  Ext Struct In20/1 -> Bus Selector20/1
  Bus Selector20/1 -> Mux6/3
  Bus Selector23/1 -> Mux7/3
  Ext Struct In23/1 -> Bus Selector23/1
  Mux7/1 -> Output7/1
  Ext Struct In25/1 -> Bus Selector25/1
  Bus Selector25/1 -> Mux7/2
  Bus Selector24/1 -> Mux7/1
  Ext Struct In24/1 -> Bus Selector24/1
  Ext Struct In27/1 -> Bus Selector27/1
  Bus Selector27/1 -> Mux8/1
  Bus Selector28/1 -> Mux8/2
  Ext Struct In28/1 -> Bus Selector28/1
  Mux8/1 -> Output8/1
  Ext Struct In26/1 -> Bus Selector26/1
  Bus Selector26/1 -> Mux8/3
